simulink model "missile_core"  (R2022a)
settings: Solver=FixedStepAuto  StartTime=0.0  StopTime=10  FixedStep=0.001  RelTol=1e-3
StopFcn:
  | airframe_plot
undefined symbols (not defined in the file or in its folder): phi, r, sigbuilder_block, theta
libraries: robotgazebolib x6, simulink x1, simulink_extras x1
settings Model: Creator=amani  LastModifiedBy=amani

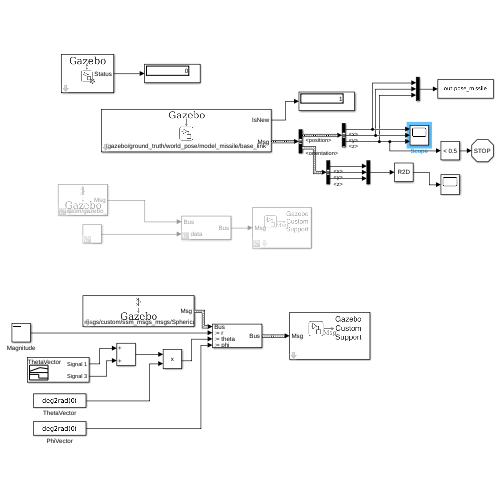
[thumbnail: Simulink's stored preview of the top-level diagram]
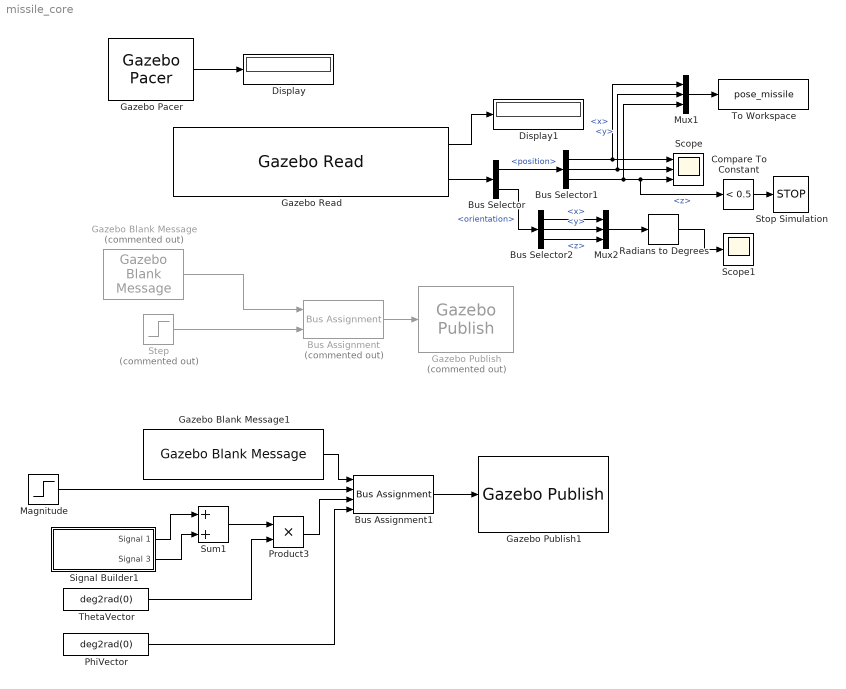
== system missile_core ==
  Bus Assignment : BusAssignment  Commented=on  AssignedSignals=data
  Bus Assignment1 : BusAssignment  AssignedSignals=r,theta,phi
  Bus Selector : BusSelector  OutputSignals=position,orientation
  Bus Selector1 : BusSelector  OutputSignals=x,y,z
  Bus Selector2 : BusSelector  OutputSignals=x,y,z
  Compare To Constant : simulink/Logic and Bit Operations/Compare To Constant  relop=<  const=0.5  OutDataTypeStr=boolean
  Display : Display
  Display1 : Display
  Gazebo Blank Message : robotgazebolib/Gazebo Blank Message  Commented=on  msgType=gazebo_msgs/custom/gazebo_msgs/Double  sampleTime=0.001  busName='Gazebo_SL_Bus_gazebo_msgs_custom_gazebo_msgs_Double'
      settings: SourceProductBaseCode=RO
  Gazebo Blank Message1 : robotgazebolib/Gazebo Blank Message  msgType=gazebo_msgs/custom/ssm_msgs_msgs/SphericalVector  sampleTime=0.001  busName='Gazebo_SL_Bus_gazebo_msgs_custom_ssm_msgs_msgs_SphericalVector'
      settings: SourceProductBaseCode=RO
  Gazebo Pacer : robotgazebolib/Gazebo Pacer  ResetBehavior=Reset Gazebo simulation time and scene  SampleTime=0.001
      settings: SourceProductBaseCode=RO
  Gazebo Publish : robotgazebolib/Gazebo Publish  Commented=on  topicSource=Specify your own  topic=/gazebo/my_world/booster_force  messageType=gazebo_msgs/custom/gazebo_msgs/Double  sampleTime=0.001
      settings: SourceProductBaseCode=RO
  Gazebo Publish1 : robotgazebolib/Gazebo Publish  topicSource=Specify your own  topic=/gazebo/my_world/thrust_force  messageType=gazebo_msgs/custom/ssm_msgs_msgs/SphericalVector  sampleTime=0.001
      settings: SourceProductBaseCode=RO
  Gazebo Read : robotgazebolib/Gazebo Read  topicSource=From Gazebo  topic=/gazebo/ground_truth/world_pose/model_missile/base_link  messageType=gazebo_msgs/Pose  sampleTime=0.001
      settings: SourceProductBaseCode=RO
  Magnitude : Step  Time=3  Before=5.9659e+03  After=0  SampleTime=0
  Mux1 : Mux  Inputs=3
  Mux2 : Mux  Inputs=3
  PhiVector : Constant  Value=deg2rad(0)
  Product3 : Product
  Radians to Degrees : simulink_extras/Transformations/Radians to Degrees
  Scope : Scope  NumInputPorts=3
  Scope1 : Scope
  Signal Builder1 : Subsystem  Tag=STV Subsys  LoadFcn=sigbuilder_block('load');  StartFcn=sigbuilder_block('start');  StopFcn=sigbuilder_block('stop');  ClipboardFcn=sigbuilder_block('clipboard');  mask(Sigbuilder block){tuvar=[0:10]}
      mask help: Simulink:masks:SigbuilderBlock_MD
      mask init:
      | if ~strcmp(get_param(bdroot(gcbh),'SimulationStatus'),'stopped') tuvar = sigbuilder_block('maskInit'); end
      settings: CopyFcn=sigbuilder_block('copy');  DeleteFcn=sigbuilder_block('delete');  ModelCloseFcn=sigbuilder_block('modelClose');  PreSaveFcn=sigbuilder_block('preSave');  PauseFcn=sigbuilder_block('pause');  ContinueFcn=sigbuilder_block('continue');  NameChangeFcn=sigbuilder_block('namechange');  OpenFcn=sigbuilder_block('open',[40.5 0 1422 705 ]);  CloseFcn=sigbuilder_block('close');
      mask Display: plot(0, 0, 100, 100,[2, 2, 32, 32, 2], [68, 8, 8, 68, 68],[32, 2], [38, 38], [32, 19, 2],[53, 60, 44], [32, 17, 17, 2],[16, 16, 31, 31]);txt = getActiveGroup(gcbh);text(2, 100, txt,'verticalAlignment', 'top');
  Step : Step  Commented=on  Time=5  Before=780*9.8  After=0  SampleTime=0
  Stop Simulation : Stop
  Sum1 : Sum
  ThetaVector : Constant  Value=deg2rad(0)
  To Workspace : ToWorkspace  VariableName=pose_missile  SaveFormat=Structure With Time  SampleTime=-1
  wires:
  Gazebo Pacer/1 -> Display/1
  Bus Assignment/1 -> Gazebo Publish/1
  Gazebo Blank Message/1 -> Bus Assignment/1
  Step/1 -> Bus Assignment/2
  Gazebo Read/1 -> Display1/1
  Gazebo Read/2 -> Bus Selector/1
  Bus Selector/1 -> Bus Selector1/1  "<position>"
  Bus Selector1/1 -> Mux1/1, Scope/1  "<x>"
  Bus Selector1/2 -> Mux1/2, Scope/2  "<y>"
  Bus Selector1/3 -> Mux1/3, Compare To Constant/1, Scope/3  "<z>"
  Compare To Constant/1 -> Stop Simulation/1
  Gazebo Blank Message1/1 -> Bus Assignment1/1
  Bus Assignment1/1 -> Gazebo Publish1/1
  Magnitude/1 -> Bus Assignment1/2
  Product3/1 -> Bus Assignment1/3
  Signal Builder1/2(Signal 3) -> Sum1/2
  Sum1/1 -> Product3/1
  ThetaVector/1 -> Product3/2
  Signal Builder1/1(Signal 1) -> Sum1/1
  PhiVector/1 -> Bus Assignment1/4
  Radians to Degrees/1 -> Scope1/1
  Mux1/1 -> To Workspace/1
  Mux2/1 -> Radians to Degrees/1
  Bus Selector/2 -> Bus Selector2/1  "<orientation>"
  Bus Selector2/1 -> Mux2/1  "<x>"
  Bus Selector2/2 -> Mux2/2  "<y>"
  Bus Selector2/3 -> Mux2/3  "<z>"

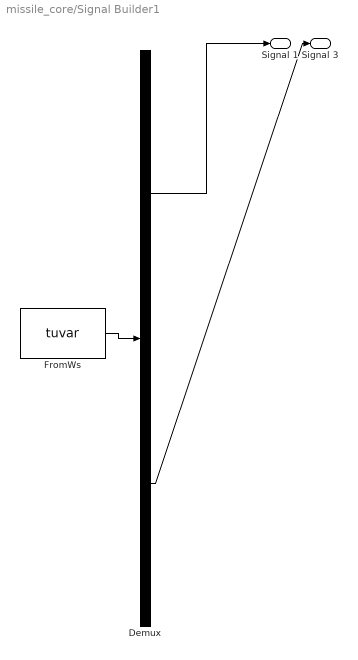
== system missile_core/Signal Builder1 ==
  Demux : Demux  Tag=STV Demux  Outputs=2
      settings: DisplayOption=none
  FromWs : FromWorkspace  Tag=STV FromWs  VariableName=tuvar
      SigBuilderData=|
      | common.afterFinalStr = 'Extrapolate'
      | common.sampleTime = 0
      | dataSet.timeRange = [0 60]
      | dataSet.name = 'ThetaVector'
      | sbobj.Groups.Name = 'ThetaVector'
      | sbobj.Groups.Signals(1).Name = 'Signal 1'
      | sbobj.Groups.Signals(1).XData = [0 1 2 3 60]
      | sbobj.Groups.Signals(1).YData = [0 0 1 0 0]
      | sbobj.Groups.Signals(2).Name = 'Signal 3'
      | sbobj.Groups.Signals(2).XData = [0 3 4 5 60]
      | sbobj.Groups.Signals(2).YData = [0 0 -2 0 0]
      | sbobj.Groups.TimeRange = [0 60]
  Signal 1 : Outport  Tag=STV Outport
  Signal 3 : Outport  Tag=STV Outport  Port=2
  wires:
  FromWs/1 -> Demux/1
  Demux/1 -> Signal 1/1
  Demux/2 -> Signal 3/1
